simulink model "Lab_1_52"  (R2025b)
settings: Solver=ode4  StartTime=0.0  StopTime=60  FixedStep=0.2  MaxStep=0  MinStep=1  RelTol=1e-3
settings Model: Creator=james  LastModifiedBy=james
settings DataIOCC: ReturnWorkspaceOutputs=off

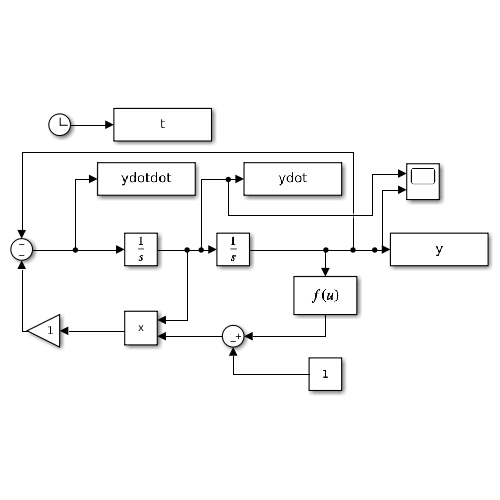
[thumbnail: Simulink's stored preview of the top-level diagram]
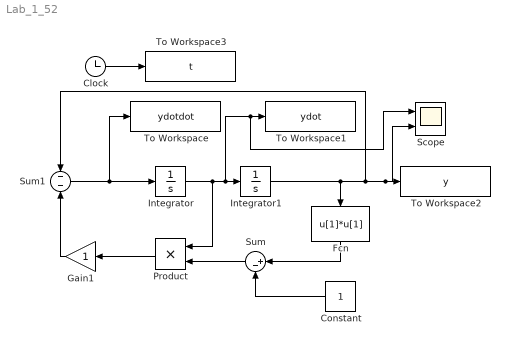
== system Lab_1_52 ==
  Clock : Clock
  Constant : Constant
  Fcn : Fcn  Expr=u[1]*u[1]
  Gain1 : Gain
  Integrator : Integrator  InitialCondition=0.5
  Integrator1 : Integrator  InitialCondition=-0.5
  Product : Product
  Scope : Scope  NumInputPorts=2
      settings: ActiveDisplayYMinimum=-3.3440872923691023  ActiveDisplayYMaximum=3.3430478496592735
  Sum : Sum  Inputs=|+-
  Sum1 : Sum  Inputs=--
  To Workspace : ToWorkspace  VariableName=ydotdot  SampleTime=-1
  To Workspace1 : ToWorkspace  VariableName=ydot  SampleTime=-1
  To Workspace2 : ToWorkspace  VariableName=y  SampleTime=-1
  To Workspace3 : ToWorkspace  VariableName=t  SaveFormat=Timeseries  SampleTime=-1
  wires:
  Clock/1 -> To Workspace3/1
  Fcn/1 -> Sum/1
  Constant/1 -> Sum/2
  Sum/1 -> Product/2
  Product/1 -> Gain1/1
  Gain1/1 -> Sum1/2
  Sum1/1 -> To Workspace/1, Integrator/1
  Integrator/1 -> Product/1, Scope/1, To Workspace1/1, Integrator1/1
  Integrator1/1 -> Sum1/1, Scope/2, To Workspace2/1, Fcn/1
